simulink model "model"  (R2019b)
settings: Solver=VariableStepAuto  StartTime=0.0  StopTime=20  RelTol=1e-3
values from neighbouring files (symbols this model uses):
  A = 0.0654    [config.m]
  AirDensity = 1.2041    [config.m]
  Ca = 0.28    [config.m]
  Cw = 0.2    [config.m]
  DegreePerSecond = 60/0.14    (= 428.571428571)    [config.m]
  HeadingPerSecondPerDegree = 0.5    [config.m]
  KV = 900    [config.m]
  MotorSpoolUpTime = 0.2    [config.m]
  PlaneMass = 1.117 + 0.506 + 2*0.192    (= 2.007)    [config.m]
  PropAngle = 4.5 * 0.0254    (= 0.1143)    [config.m]
  PropEff = 0.7    [config.m]
  PropRadius = 10/2 * 0.0254    (= 0.127)    [config.m]
  T_Roll = 0.1    [config.m]
  WingArea = 0.3    [config.m]
libraries: simulink x7
settings Model: Creator=paul  LastModifiedBy=paul
settings SolverCC: ZeroCrossAlgorithm=Adaptive
settings DataIOCC: ReturnWorkspaceOutputs=off
settings DebuggingCC: MaxConsecutiveZCsMsg=none  ArithmeticOperatorsInVariantConditions=warning
settings SFSimCC: SimUseLocalCustomCode=off  CustomCodeUndefinedFunction=UseInterfaceOnly
settings RTWCC: RTWUseLocalCustomCode=off

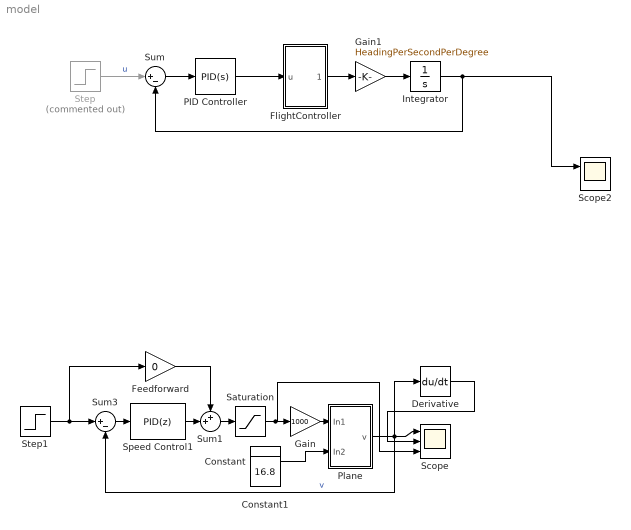
== system model ==
  Constant : Constant  Value=16.8
  Constant1 : Constant  Value=16.8
  Derivative : Derivative
  "Feedforward " : Gain  Gain=0
  FlightController : Subsystem
  Gain : Gain  Gain=1000
  Gain1 : Gain  Gain=HeadingPerSecondPerDegree
  Integrator : Integrator
  PID Controller : simulink/Continuous/PID Controller  Controller=PID  Form=Parallel  TimeDomain=Continuous-time  SampleTime=-1  IntegratorMethod=Forward Euler  FilterMethod=Forward Euler  ControllerParametersSource=internal  P=1.5  I=0  D=0  UseFilter=on  N=100  TunerSelectOption=Transfer Function Based (PID Tuner App)  InitialConditionSource=internal  InitialConditionForIntegrator=0  InitialConditionForFilter=0  DifferentiatorICPrevScaledInput=0  ExternalReset=none  TrackingMode=off  Kt=1  LimitOutput=off  UpperSaturationLimit=inf  LowerSaturationLimit=-inf  LinearizeAsGain=on  AntiWindupMode=none  Kb=1  POutMin=[]  POutMax=[]  IOutMin=[]  IOutMax=[]  DOutMin=[]  DOutMax=[]  NOutMin=[]  NOutMax=[]  SumOutMin=[]  SumOutMax=[]  SaturationOutMin=[]  SaturationOutMax=[]  PParamMin=[]  PParamMax=[]  IParamMin=[]  IParamMax=[]  DParamMin=[]  DParamMax=[]  NParamMin=[]  NParamMax=[]  KbParamMin=[]  KbParamMax=[]  KtParamMin=[]  KtParamMax=[]  KbOutMin=[]  KbOutMax=[]  KtOutMin=[]  KtOutMax=[]  IntegratorOutMin=[]  IntegratorOutMax=[]  FilterOutMin=[]  FilterOutMax=[]  SumI1OutMin=[]  SumI1OutMax=[]  SumI2OutMin=[]  SumI2OutMax=[]  SumI3OutMin=[]  SumI3OutMax=[]  SumI4OutMin=[]  SumI4OutMax=[]  SumDOutMin=[]  SumDOutMax=[]  DifferentiatorOutMin=[]  DifferentiatorOutMax=[]  FilterDiffOutCoefMin=[]  FilterDiffOutCoefMax=[]  ReciprocalOutMin=[]  ReciprocalOutMax=[]  SumDenOutMin=[]  SumDenOutMax=[]  SumNumOutMin=[]  SumNumOutMax=[]  DivideOutMin=[]  DivideOutMax=[]  IntegratorContinuousStateAttributes=''  IntegratorStateMustResolveToSignalObject=off  IntegratorRTWStateStorageClass=Auto  FilterContinuousStateAttributes=''  FilterStateMustResolveToSignalObject=off  FilterRTWStateStorageClass=Auto  ParallelPVariant=InternalParameters  IdealPVariant=Disabled  IVariant=InternalParameters  DVariant=InternalParameters  IntegratorVariant=Continuous  SatVariant=Disabled  AWVariant=Passthrough  PCopyVariant=Disabled  TRVariant=Disabled  FdbkBlocksVariant=Forward  IdealPFdbkVariant=Disabled  SatFdbkVariant=Disabled  DerivativeFilterVariant=ContFilter  NVariant=InternalParameters  NCopyVariant=Disabled  FilterICVariant=InternalICsFilter  IntegratorICVariant=InternalICs  ExternalResetVariant=Disabled  TRSumVariant=Passthrough  SumFdbkVariant=Disabled  SumVariant=Sum_PID
  Plane : Subsystem
  Saturation : Saturate  UpperLimit=1  LowerLimit=0
  Scope : Scope  NumInputPorts=3
  Scope2 : Scope  NumInputPorts=2
  Speed Control1 : simulink/Continuous/PID Controller  Controller=PID  Form=Parallel  TimeDomain=Discrete-time  SampleTime=0.1  IntegratorMethod=Forward Euler  FilterMethod=Forward Euler  ControllerParametersSource=internal  P=1  I=0  D=0  UseFilter=on  N=100  TunerSelectOption=Transfer Function Based (PID Tuner App)  ZeroCross=off  InitialConditionSource=internal  InitialConditionForIntegrator=0  InitialConditionForFilter=0  DifferentiatorICPrevScaledInput=0  ExternalReset=none  TrackingMode=off  Kt=1  LimitOutput=off  UpperSaturationLimit=1  LowerSaturationLimit=0  LinearizeAsGain=off  AntiWindupMode=none  Kb=1  POutMin=[]  POutMax=[]  IOutMin=[]  IOutMax=[]  DOutMin=[]  DOutMax=[]  NOutMin=[]  NOutMax=[]  SumOutMin=[]  SumOutMax=[]  SaturationOutMin=[]  SaturationOutMax=[]  PParamMin=[]  PParamMax=[]  IParamMin=[]  IParamMax=[]  DParamMin=[]  DParamMax=[]  NParamMin=[]  NParamMax=[]  KbParamMin=[]  KbParamMax=[]  KtParamMin=[]  KtParamMax=[]  KbOutMin=[]  KbOutMax=[]  KtOutMin=[]  KtOutMax=[]  IntegratorOutMin=[]  IntegratorOutMax=[]  FilterOutMin=[]  FilterOutMax=[]  SumI1OutMin=[]  SumI1OutMax=[]  SumI2OutMin=[]  SumI2OutMax=[]  SumI3OutMin=[]  SumI3OutMax=[]  SumI4OutMin=[]  SumI4OutMax=[]  SumDOutMin=[]  SumDOutMax=[]  DifferentiatorOutMin=[]  DifferentiatorOutMax=[]  FilterDiffOutCoefMin=[]  FilterDiffOutCoefMax=[]  ReciprocalOutMin=[]  ReciprocalOutMax=[]  SumDenOutMin=[]  SumDenOutMax=[]  SumNumOutMin=[]  SumNumOutMax=[]  DivideOutMin=[]  DivideOutMax=[]  IntegratorContinuousStateAttributes=''  IntegratorStateMustResolveToSignalObject=off  IntegratorRTWStateStorageClass=Auto  FilterContinuousStateAttributes=''  FilterStateMustResolveToSignalObject=off  FilterRTWStateStorageClass=Auto  ParallelPVariant=InternalParameters  IdealPVariant=Disabled  IVariant=InternalParameters  DVariant=InternalParameters  IntegratorVariant=Discrete  SatVariant=Disabled  AWVariant=Passthrough  PCopyVariant=Disabled  TRVariant=Disabled  FdbkBlocksVariant=Forward  IdealPFdbkVariant=Disabled  SatFdbkVariant=Disabled  DerivativeFilterVariant=ForwardEulerFilter  NVariant=InternalParameters  NCopyVariant=Disabled  FilterICVariant=InternalICsFilter  IntegratorICVariant=InternalICs  ExternalResetVariant=Disabled  TRSumVariant=Passthrough  SumFdbkVariant=Disabled  SumVariant=Sum_PID
  Step : Step  Commented=on  Time=0  After=90  SampleTime=0
  Step1 : Step  Time=10  Before=1000  After=0  SampleTime=0
  Sum : Sum  Inputs=|+-
  Sum1 : Sum  Inputs=++|
  Sum3 : Sum  Inputs=|+-
  wires:
  Constant/1 -> Plane/2(In2)
  Plane/1(v) -> Derivative/1, Sum3/2, Scope/1  "v"
  Step1/1 -> Sum3/1, "Feedforward "/1
  Gain/1 -> Plane/1(In1)
  Integrator/1 -> Scope2/1, Sum/2
  Step/1 -> Sum/1  "u"
  Sum/1 -> PID Controller/1
  PID Controller/1 -> FlightController/1(u)
  Gain1/1 -> Integrator/1
  FlightController/1(Out1) -> Gain1/1
  "Feedforward "/1 -> Sum1/1
  Speed Control1/1 -> Sum1/2
  Sum3/1 -> Speed Control1/1
  Sum1/1 -> Saturation/1
  Saturation/1 -> Scope/3, Gain/1
  Derivative/1 -> Scope/2

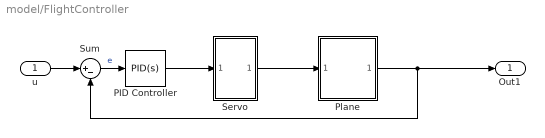
== system model/FlightController ==
  u : Inport
  PID Controller : simulink/Continuous/PID Controller  Controller=PID  Form=Parallel  TimeDomain=Continuous-time  SampleTime=-1  IntegratorMethod=Forward Euler  FilterMethod=Forward Euler  ControllerParametersSource=internal  P=60  I=0  D=10  UseFilter=on  N=100  TunerSelectOption=Transfer Function Based (PID Tuner App)  InitialConditionSource=internal  InitialConditionForIntegrator=0  InitialConditionForFilter=0  DifferentiatorICPrevScaledInput=0  ExternalReset=none  TrackingMode=off  Kt=1  LimitOutput=off  UpperSaturationLimit=inf  LowerSaturationLimit=-inf  LinearizeAsGain=on  AntiWindupMode=none  Kb=1  POutMin=[]  POutMax=[]  IOutMin=[]  IOutMax=[]  DOutMin=[]  DOutMax=[]  NOutMin=[]  NOutMax=[]  SumOutMin=[]  SumOutMax=[]  SaturationOutMin=[]  SaturationOutMax=[]  PParamMin=[]  PParamMax=[]  IParamMin=[]  IParamMax=[]  DParamMin=[]  DParamMax=[]  NParamMin=[]  NParamMax=[]  KbParamMin=[]  KbParamMax=[]  KtParamMin=[]  KtParamMax=[]  KbOutMin=[]  KbOutMax=[]  KtOutMin=[]  KtOutMax=[]  IntegratorOutMin=[]  IntegratorOutMax=[]  FilterOutMin=[]  FilterOutMax=[]  SumI1OutMin=[]  SumI1OutMax=[]  SumI2OutMin=[]  SumI2OutMax=[]  SumI3OutMin=[]  SumI3OutMax=[]  SumI4OutMin=[]  SumI4OutMax=[]  SumDOutMin=[]  SumDOutMax=[]  DifferentiatorOutMin=[]  DifferentiatorOutMax=[]  FilterDiffOutCoefMin=[]  FilterDiffOutCoefMax=[]  ReciprocalOutMin=[]  ReciprocalOutMax=[]  SumDenOutMin=[]  SumDenOutMax=[]  SumNumOutMin=[]  SumNumOutMax=[]  DivideOutMin=[]  DivideOutMax=[]  IntegratorContinuousStateAttributes=''  IntegratorStateMustResolveToSignalObject=off  IntegratorRTWStateStorageClass=Auto  FilterContinuousStateAttributes=''  FilterStateMustResolveToSignalObject=off  FilterRTWStateStorageClass=Auto  ParallelPVariant=InternalParameters  IdealPVariant=Disabled  IVariant=InternalParameters  DVariant=InternalParameters  IntegratorVariant=Continuous  SatVariant=Disabled  AWVariant=Passthrough  PCopyVariant=Disabled  TRVariant=Disabled  FdbkBlocksVariant=Forward  IdealPFdbkVariant=Disabled  SatFdbkVariant=Disabled  DerivativeFilterVariant=ContFilter  NVariant=InternalParameters  NCopyVariant=Disabled  FilterICVariant=InternalICsFilter  IntegratorICVariant=InternalICs  ExternalResetVariant=Disabled  TRSumVariant=Passthrough  SumFdbkVariant=Disabled  SumVariant=Sum_PID
  Plane : Subsystem
  Servo : Subsystem
  Sum : Sum  Inputs=|+-
  Out1 : Outport  VectorParamsAs1DForOutWhenUnconnected=off
  wires:
  Sum/1 -> PID Controller/1  "e"
  u/1 -> Sum/1
  Plane/1(angle) -> Sum/2, Out1/1
  PID Controller/1 -> Servo/1(In1)
  Servo/1(Out1) -> Plane/1(servo)

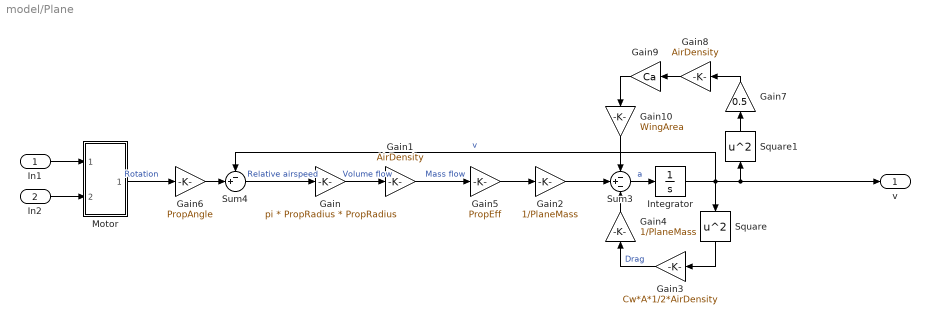
== system model/Plane ==
  In1 : Inport
  In2 : Inport  Port=2
  Gain : Gain  Gain=pi * PropRadius * PropRadius
  Gain1 : Gain  Gain=AirDensity
  Gain10 : Gain  Gain=WingArea
  Gain2 : Gain  Gain=1/PlaneMass
  Gain3 : Gain  Gain=Cw*A*1/2*AirDensity
  Gain4 : Gain  Gain=1/PlaneMass
  Gain5 : Gain  Gain=PropEff
  Gain6 : Gain  Gain=PropAngle
  Gain7 : Gain  Gain=0.5
  Gain8 : Gain  Gain=AirDensity
  Gain9 : Gain  Gain=Ca
  Integrator : Integrator
  Motor : Subsystem
  Square : Math  Operator=square  SaturateOnIntegerOverflow=on
  Square1 : Math  Operator=square  SaturateOnIntegerOverflow=on
  Sum3 : Sum  Inputs=-+-
  Sum4 : Sum  Inputs=-+|
  v : Outport  VectorParamsAs1DForOutWhenUnconnected=off
  wires:
  Gain5/1 -> Gain2/1
  Gain1/1 -> Gain5/1  "Mass flow"
  Gain4/1 -> Sum3/3
  In2/1 -> Motor/2(V_Bat)
  Integrator/1 -> v/1, Square1/1, Sum4/1, Square/1  "v"
  Sum4/1 -> Gain/1  "Relative airspeed"
  Gain6/1 -> Sum4/2
  Motor/1(Out1) -> Gain6/1  "Rotation"
  Square/1 -> Gain3/1
  In1/1 -> Motor/1("PPM ")
  Sum3/1 -> Integrator/1  "a"
  Gain3/1 -> Gain4/1  "Drag"
  Gain/1 -> Gain1/1  "Volume flow"
  Gain2/1 -> Sum3/2
  Square1/1 -> Gain7/1
  Gain7/1 -> Gain8/1
  Gain8/1 -> Gain9/1
  Gain10/1 -> Sum3/1
  Gain9/1 -> Gain10/1

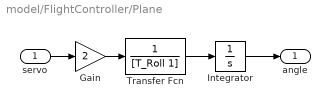
== system model/FlightController/Plane ==
  servo : Inport
  Gain : Gain  Gain=2
  Integrator : Integrator
  Transfer Fcn : TransferFcn  Denominator=[T_Roll 1]
  angle : Outport  VectorParamsAs1DForOutWhenUnconnected=off
  wires:
  Gain/1 -> Transfer Fcn/1
  servo/1 -> Gain/1
  Transfer Fcn/1 -> Integrator/1
  Integrator/1 -> angle/1

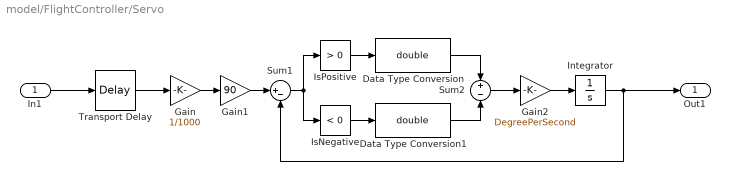
== system model/FlightController/Servo ==
  In1 : Inport
  Data Type Conversion : DataTypeConversion  OutDataTypeStr=double
  Data Type Conversion1 : DataTypeConversion  OutDataTypeStr=double
  Gain : Gain  Gain=1/1000
  Gain1 : Gain  Gain=90
  Gain2 : Gain  Gain=DegreePerSecond
  Integrator : Integrator  LimitOutput=on  UpperSaturationLimit=90  LowerSaturationLimit=-90
  IsNegative : simulink/Logic and Bit Operations/Compare To Zero  relop=<  OutDataTypeStr=boolean
  IsPositive : simulink/Logic and Bit Operations/Compare To Zero  relop=>  OutDataTypeStr=boolean
  Sum1 : Sum  Inputs=|+-
  Sum2 : Sum  Inputs=+|-
  Transport Delay : TransportDelay  DelayTime=0.01
  Out1 : Outport  VectorParamsAs1DForOutWhenUnconnected=off
  wires:
  In1/1 -> Transport Delay/1
  Gain1/1 -> Sum1/1
  Gain/1 -> Gain1/1
  Sum1/1 -> IsNegative/1, IsPositive/1
  Data Type Conversion/1 -> Sum2/1
  Integrator/1 -> Out1/1, Sum1/2
  Data Type Conversion1/1 -> Sum2/2
  IsPositive/1 -> Data Type Conversion/1
  Gain2/1 -> Integrator/1
  IsNegative/1 -> Data Type Conversion1/1
  Sum2/1 -> Gain2/1
  Transport Delay/1 -> Gain/1

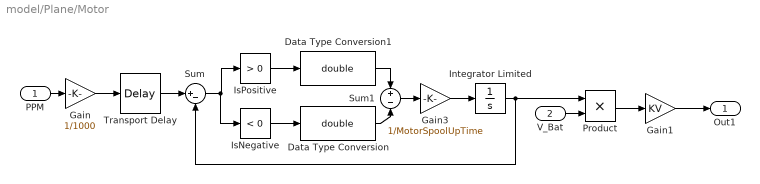
== system model/Plane/Motor ==
  "PPM " : Inport
  V_Bat : Inport  Port=2
  Data Type Conversion : DataTypeConversion  OutDataTypeStr=double
  Data Type Conversion1 : DataTypeConversion  OutDataTypeStr=double
  Gain : Gain  Gain=1/1000
  Gain1 : Gain  Gain=KV
  Gain3 : Gain  Gain=1/MotorSpoolUpTime
  Integrator Limited : Integrator  LimitOutput=on  UpperSaturationLimit=1  LowerSaturationLimit=0
  IsNegative : simulink/Logic and Bit Operations/Compare To Zero  relop=<  OutDataTypeStr=boolean
  IsPositive : simulink/Logic and Bit Operations/Compare To Zero  relop=>  OutDataTypeStr=boolean
  Product : Product
  Sum : Sum  Inputs=|+-
  Sum1 : Sum  Inputs=+|-
  Transport Delay : TransportDelay  DelayTime=0.01
  Out1 : Outport  VectorParamsAs1DForOutWhenUnconnected=off
  wires:
  IsNegative/1 -> Data Type Conversion/1
  IsPositive/1 -> Data Type Conversion1/1
  Sum/1 -> IsNegative/1, IsPositive/1
  V_Bat/1 -> Product/2
  Sum1/1 -> Gain3/1
  Product/1 -> Gain1/1
  Gain1/1 -> Out1/1
  Data Type Conversion1/1 -> Sum1/1
  Data Type Conversion/1 -> Sum1/2
  "PPM "/1 -> Gain/1
  Gain/1 -> Transport Delay/1
  Integrator Limited/1 -> Product/1, Sum/2
  Transport Delay/1 -> Sum/1
  Gain3/1 -> Integrator Limited/1
